simulink model "test_controler"  (R2015a)
settings: Solver=FixedStepDiscrete  StartTime=0.0  StopTime=10.0  RelTol=1e-3
values from neighbouring files (symbols this model uses):
  K = Kn(1:4)    [teste_integrador.m]
  Nbar = 0    [teste_integrador.m]
  Nx = N(1:4,:)    [teste_integrador.m]
undefined symbols (not defined in the file or in its folder): T
settings Model: Creator=alunos  LastModifiedBy=hdplsa
settings DataIOCC: LimitDataPoints=off

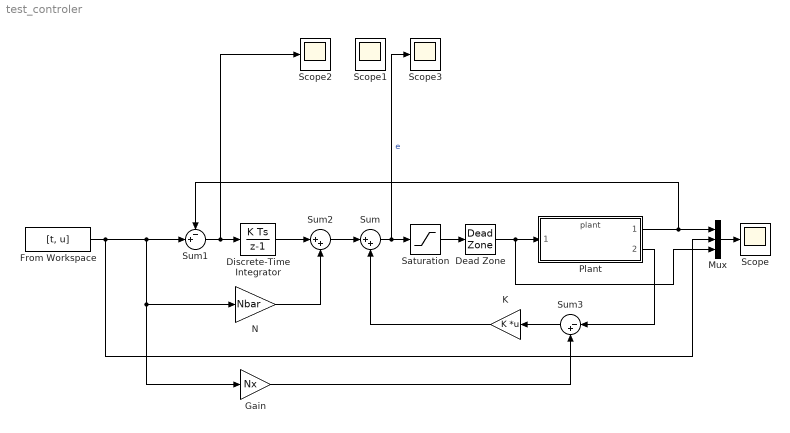
== system test_controler ==
  Dead Zone : DeadZone  LowerValue=-0.17  UpperValue=0.45  SaturateOnIntegerOverflow=on
  Discrete-Time Integrator : DiscreteIntegrator  gainval=Ki  InitialConditionSetting=State (most efficient)  SampleTime=-1
  From Workspace : FromWorkspace  VariableName=[t, u]  SampleTime=T
  Gain : Gain  Gain=Nx
  K : Gain  Gain=K  Multiplication=Matrix(K*u)
  Mux : Mux  Inputs=3
  N : Gain  Gain=Nbar
  Plant : ModelReference  ModelNameDialog=plant.slx  SimulationMode=Normal  ModelReferenceVersion=1.20  CopyOfModelName=plant.slx  DefaultDataLogging=on
  Saturation : Saturate  UpperLimit=5*2*pi  LowerLimit=-5*2*pi
  Scope{,1..3} (4 alike) : Scope
      Scope settings: SaveName=test_controller
      Scope1 settings: SaveName=test_controller1
      Scope2 settings: SaveName=test_controller2
      Scope3 settings: SaveName=test_controller3
  Sum : Sum  Inputs=|++
  Sum1 : Sum  Inputs=-+|
  Sum2 : Sum  Inputs=|++
  Sum3 : Sum  Inputs=|-+
  wires:
  K/1 -> Sum/2
  Plant/1 -> Mux/1, Sum1/1
  Mux/1 -> Scope/1
  Saturation/1 -> Dead Zone/1
  Dead Zone/1 -> Mux/3, Plant/1
  Sum/1 -> Scope3/1, Saturation/1  "e"
  Sum1/1 -> Discrete-Time Integrator/1, Scope2/1
  From Workspace/1 -> Gain/1, N/1, Sum1/2, Mux/2
  Discrete-Time Integrator/1 -> Sum2/1
  N/1 -> Sum2/2
  Sum2/1 -> Sum/1
  Sum3/1 -> K/1
  Plant/2 -> Sum3/1
  Gain/1 -> Sum3/2
